simulink model "SF017A_HiLoadStallLimr"  (R2013b)
settings: Solver=FixedStepDiscrete  StartTime=0.0  StopTime=1  FixedStep=.002  RelTol=1e-3
values from neighbouring files (symbols this model uses):
  ARCHGLBPRM_2MILLISEC_SEC_F32 = DataDict.Constant    [SF017A_HiLoadStallLimr_DataDict.m]
  HiLoadStallLimrMotVelMgnThd = DataDict.Calibration    [SF017A_HiLoadStallLimr_DataDict.m]
  HiLoadStallLimrStallMotTqCmdLimY = DataDict.Calibration    [SF017A_HiLoadStallLimr_DataDict.m]
  HiLoadStallLimrStallMotTqLimSlewRate = DataDict.Calibration    [SF017A_HiLoadStallLimr_DataDict.m]
  SYSGLBPRM_MOTTQCMDHILIM_MOTNWTMTR_F32 = DataDict.Constant    [SF017A_HiLoadStallLimr_DataDict.m]
libraries: Fil x2, FixdToFloat x2, NxtrLim x2, simulink x1, FloatToFixd x1, LnrIntrpn x1
settings Model: Creator=qzwc4r  LastModifiedBy=qzwc4r
settings DataIOCC: LimitDataPoints=off  SaveFormat=Structure  ReturnWorkspaceOutputs=on
settings OptimizationCC: BlockReduction=off  InlineParams=on  ZeroExternalMemoryAtStartup=off  ZeroInternalMemoryAtStartup=off  OptimizeModelRefInitCode=on  LifeSpan=1
settings DebuggingCC: SignalInfNanChecking=error  SignalRangeChecking=warning  UnderspecifiedInitializationDetection=Simplified  SolverPrmCheckMsg=error  InheritedTsInSrcMsg=error  DiscreteInheritContinuousMsg=error  SingleTaskRateTransMsg=error  TasksWithSamePriorityMsg=error  SigSpecEnsureSampleTimeMsg=error  CheckMatrixSingularityMsg=error  IntegerOverflowMsg=error  ParameterUnderflowMsg=error  ParameterPrecisionLossMsg=error  ParameterTunabilityLossMsg=error  FixptConstUnderflowMsg=warning  FixptConstOverflowMsg=warning  VectorMatrixConversionMsg=error  SignalLabelMismatchMsg=error  UnconnectedInputMsg=error  UnconnectedOutputMsg=error  UnconnectedLineMsg=error  SFcnCompatibilityMsg=error  UniqueDataStoreMsg=warning  BusObjectLabelMismatch=error  RootOutportRequireBusObject=error  AssertControl=DisableAll  ModelReferenceIOMsg=error  ModelReferenceVersionMismatchMessage=warning  ModelReferenceIOMismatchMessage=error  ModelReferenceCSMismatchMessage=warning  ModelReferenceDataLoggingMessage=error  StateNameClashWarn=warning  StrictBusMsg=ErrorOnBusTreatedAsVector  NonBusSignalsTreatedAsBus=error  SFUnexpectedBacktrackingDiag=error  SFInvalidInputDataAccessInChartInitDiag=error  SFNoUnconditionalDefaultTransitionDiag=error  SFTransitionOutsideNaturalParentDiag=error  SFUnconditionalTransitionShadowingDiag=error  SFUndirectedBroadcastEventsDiag=error
settings ModelReferenceCC: ModelReferenceNumInstancesAllowed=Single
settings RTWCC: SystemTargetFile=autosar.tlc  GenCodeOnly=on  TemplateMakefile=ert_default_tmf  Description=AUTOSAR  GenerateReport=on  ProcessScript=autosar_make_rtw_hook  LaunchReport=on
settings CodeAppCC: GenerateComments=off  IgnoreCustomStorageClasses=off  CustomSymbolStrType=$N$R$M  CustomSymbolStrBlkIO=$N$M  SimulinkBlockComments=off
settings STFCustomTargetCC: ParMdlRefBuildCompliant=on  CompOptLevelCompliant=on  IncludeMdlTerminateFcn=off  CombineOutputUpdateFcns=on  SuppressErrorStatus=on  ERTFirstTimeCompliant=on  ERTCustomFileBanners=on  SupportNonFinite=off  SupportComplex=off  SupportContinuousTime=off  SupportNonInlinedSFcns=off  MATLABClassNameForMDSCustomization=Simulink.SoftwareTarget.ERTCustomization  AutosarCompliant=on  GRTInterface=off  SystemTargetFile=autosar.tlc
settings ERTTargetCC: CodeReplacementLibrary=ANSI_C  ConcurrentExecutionCompliant=off  IncludeMdlTerminateFcn=off  SuppressErrorStatus=on  SupportNonFinite=off  SupportComplex=off  ModelStepFunctionPrototypeControlCompliant=off  CPPClassGenCompliant=off  AutosarCompliant=on  InlinedParameterPlacement=NonHierarchical  ERTCustomFileTemplate=example_file_process.tlc  EnableUserReplacementTypes=on

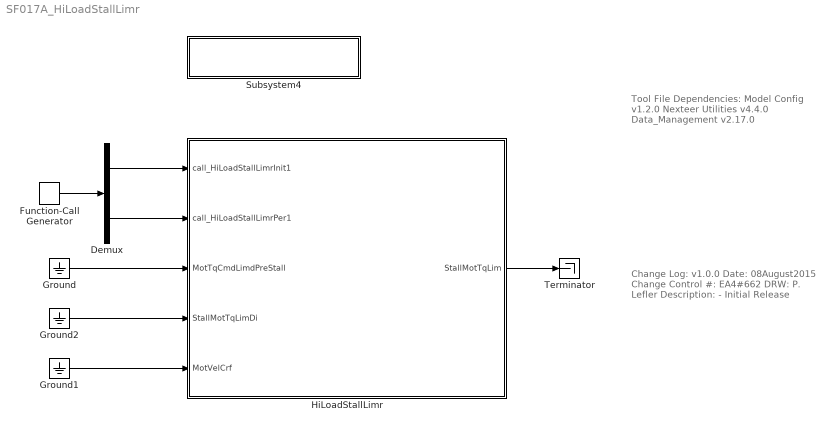
== system SF017A_HiLoadStallLimr ==
  note: Tool File Dependencies:
      |
      | Model Config v1.2.0
      | Nexteer Utilities v4.4.0
      | Data_Management v2.17.0
  note: Change Log:
      |
      | v1.0.0
      | Date: 08August2015
      | Change Control #: EA4#662
      | DRW: P. Lefler
      | Description:
      | - Initial Release
  Demux : Demux  Outputs=2
  Function-Call Generator : simulink/Ports & Subsystems/Function-Call Generator  sample_time=Ts  numberOfIterations=1
  Ground : Ground
  Ground1 : Ground
  Ground2 : Ground
  HiLoadStallLimr : Subsystem
  Subsystem4 : Subsystem  Description=|  mask(Copyright Information){none=on}
      | Copyright info block.                                               
      |                                                                     
      | Place copyright information at the top of every subsystem in design.
      mask prompts: none "No parameters"
      mask help: Place copyright information at the top of every subsystem in design.
      mask Display:
      | NxtrConf = 'Nexteer Confidential';
      | 
      | sys = bdroot; %handle for the current model ("system")
      | first = get_param(sys,'Created');
      | first = first(end-3:end);  %year is last four digits
      | 
      | last = get_param(sys,'LastModifiedDate');
      | if isempty(last)
      |     last = datestr(now,'yyyy');
      | else
      |     last = last(end-3:end);
      | end
      | 
      | if strcmp(first,last)
      |     fprintf('%s\nCopyright  %s Nexteer',NxtrConf,first);
      | else
      |     fprintf('%s\n%s%s-%s Nexteer',NxtrConf,char(169),first,last);
      | end
  Terminator : Terminator
  wires:
  Demux/1 -> HiLoadStallLimr/1(call_HiLoadStallLimrInit1)
  Demux/2 -> HiLoadStallLimr/2(call_HiLoadStallLimrPer1)
  Function-Call Generator/1 -> Demux/1
  Ground2/1 -> HiLoadStallLimr/4(StallMotTqLimDi)
  Ground/1 -> HiLoadStallLimr/3(MotTqCmdLimdPreStall)
  Ground1/1 -> HiLoadStallLimr/5(MotVelCrf)
  HiLoadStallLimr/1(StallMotTqLim) -> Terminator/1

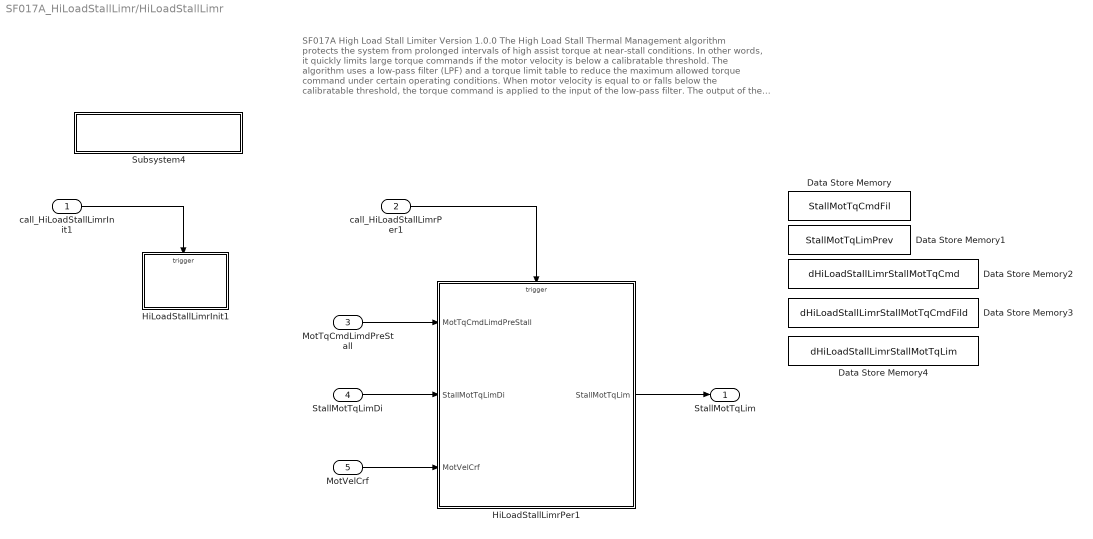
== system SF017A_HiLoadStallLimr/HiLoadStallLimr ==
  note: SF017A High Load Stall Limiter
      | Version 1.0.0
      |
      | The High Load Stall Thermal Management algorithm protects the system from prolonged intervals of high
      | assist torque at near-stall conditions. In other words, it quickly limits large torque commands if the motor
      | velocity is below a calibratable threshold.
      |      The algorithm uses a low-pass filter (LPF) and a torque limit table to reduce the maximum allowed torque
      | command under certain operating conditions. When motor velocity is equal to or falls below the calibratable
      | threshold, the torque command is applied to the input of the low-pass filter. The output of the filter ramps up
      | and indexes into the torque limit table. The output of this table is the maximum allowed torque command. A
      | slew limit calibration governs the transition rate of the table output.
  call_HiLoadStallLimrInit1 : Inport
  call_HiLoadStallLimrPer1 : Inport  Port=2
  MotTqCmdLimdPreStall : Inport  Port=3
  StallMotTqLimDi : Inport  Port=4
  MotVelCrf : Inport  Port=5
  Data Store Memory : DataStoreMemory  DataStoreName=StallMotTqCmdFil  ReadBeforeWriteMsg=warning  WriteAfterWriteMsg=warning  WriteAfterReadMsg=warning  InitialValue=[]  StateMustResolveToSignalObject=on
  Data Store Memory1 : DataStoreMemory  DataStoreName=StallMotTqLimPrev  ReadBeforeWriteMsg=warning  WriteAfterWriteMsg=warning  WriteAfterReadMsg=warning  InitialValue=[]  StateMustResolveToSignalObject=on
  Data Store Memory2 : DataStoreMemory  DataStoreName=dHiLoadStallLimrStallMotTqCmd  ReadBeforeWriteMsg=warning  WriteAfterWriteMsg=warning  WriteAfterReadMsg=warning  StateMustResolveToSignalObject=on
  Data Store Memory3 : DataStoreMemory  DataStoreName=dHiLoadStallLimrStallMotTqCmdFild  ReadBeforeWriteMsg=warning  WriteAfterWriteMsg=warning  WriteAfterReadMsg=warning  StateMustResolveToSignalObject=on
  Data Store Memory4 : DataStoreMemory  DataStoreName=dHiLoadStallLimrStallMotTqLim  ReadBeforeWriteMsg=warning  WriteAfterWriteMsg=warning  WriteAfterReadMsg=warning  StateMustResolveToSignalObject=on
  HiLoadStallLimrInit1 : Subsystem  TreatAsAtomicUnit=on
  HiLoadStallLimrPer1 : Subsystem  TreatAsAtomicUnit=on
  Subsystem4 : Subsystem  Description=|  mask(Copyright Information){none=on}
      | Copyright info block.                                               
      |                                                                     
      | Place copyright information at the top of every subsystem in design.
      mask prompts: none "No parameters"
      mask help: Place copyright information at the top of every subsystem in design.
      mask Display:
      | NxtrConf = 'Nexteer Confidential';
      | 
      | sys = bdroot; %handle for the current model ("system")
      | first = get_param(sys,'Created');
      | first = first(end-3:end);  %year is last four digits
      | 
      | last = get_param(sys,'LastModifiedDate');
      | if isempty(last)
      |     last = datestr(now,'yyyy');
      | else
      |     last = last(end-3:end);
      | end
      | 
      | if strcmp(first,last)
      |     fprintf('%s\nCopyright  %s Nexteer',NxtrConf,first);
      | else
      |     fprintf('%s\n%s%s-%s Nexteer',NxtrConf,char(169),first,last);
      | end
  StallMotTqLim : Outport
  wires:
  MotTqCmdLimdPreStall/1 -> HiLoadStallLimrPer1/1(MotTqCmdLimdPreStall)
  MotVelCrf/1 -> HiLoadStallLimrPer1/3(MotVelCrf)
  StallMotTqLimDi/1 -> HiLoadStallLimrPer1/2(StallMotTqLimDi)
  HiLoadStallLimrPer1/1(StallMotTqLim) -> StallMotTqLim/1
  call_HiLoadStallLimrPer1/1 -> HiLoadStallLimrPer1/Trigger
  call_HiLoadStallLimrInit1/1 -> HiLoadStallLimrInit1/Trigger

== system SF017A_HiLoadStallLimr/Subsystem4 ==

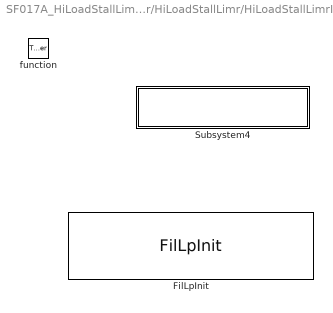
== system SF017A_HiLoadStallLimr/HiLoadStallLimr/HiLoadStallLimrInit1 ==
  function : TriggerPort  TriggerType=function-call
  FilLpInit : Fil/FilLpInit  Ic=0  Ts=ARCHGLBPRM_2MILLISEC_SEC_F32  Freq=HiLoadStallLimrMotTqCmdFilFrq  StVar=StallMotTqCmdFil
  Subsystem4 : Subsystem  Description=|  mask(Copyright Information){none=on}
      | Copyright info block.                                               
      |                                                                     
      | Place copyright information at the top of every subsystem in design.
      mask prompts: none "No parameters"
      mask help: Place copyright information at the top of every subsystem in design.
      mask Display:
      | NxtrConf = 'Nexteer Confidential';
      | 
      | sys = bdroot; %handle for the current model ("system")
      | first = get_param(sys,'Created');
      | first = first(end-3:end);  %year is last four digits
      | 
      | last = get_param(sys,'LastModifiedDate');
      | if isempty(last)
      |     last = datestr(now,'yyyy');
      | else
      |     last = last(end-3:end);
      | end
      | 
      | if strcmp(first,last)
      |     fprintf('%s\nCopyright  %s Nexteer',NxtrConf,first);
      | else
      |     fprintf('%s\n%s%s-%s Nexteer',NxtrConf,char(169),first,last);
      | end

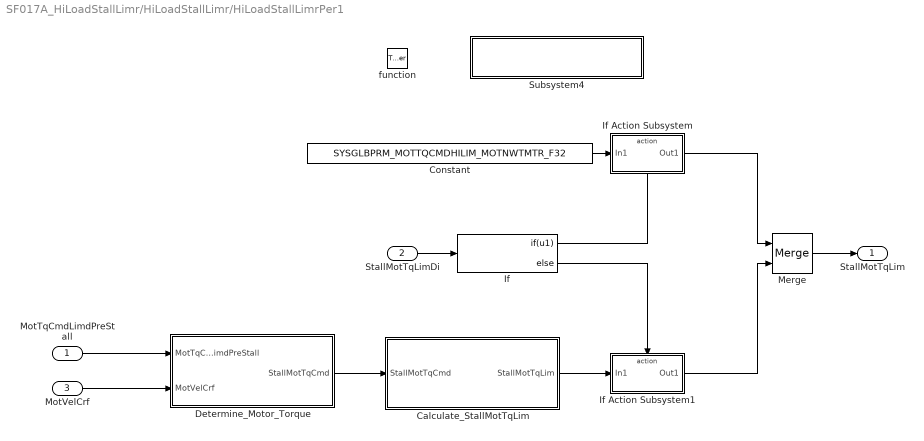
== system SF017A_HiLoadStallLimr/HiLoadStallLimr/HiLoadStallLimrPer1 ==
  MotTqCmdLimdPreStall : Inport
  StallMotTqLimDi : Inport  Port=2
  MotVelCrf : Inport  Port=3
  function : TriggerPort  TriggerType=function-call
  Calculate_StallMotTqLim : Subsystem
  Constant : Constant  Value=SYSGLBPRM_MOTTQCMDHILIM_MOTNWTMTR_F32
  Determine_Motor_Torque : Subsystem
  If : If  IfExpression=u1
  If Action Subsystem : Subsystem  TreatAsAtomicUnit=on
  If Action Subsystem1 : Subsystem  TreatAsAtomicUnit=on
  Merge : Merge
  Subsystem4 : Subsystem  Description=|  mask(Copyright Information){none=on}
      | Copyright info block.                                               
      |                                                                     
      | Place copyright information at the top of every subsystem in design.
      mask prompts: none "No parameters"
      mask help: Place copyright information at the top of every subsystem in design.
      mask Display:
      | NxtrConf = 'Nexteer Confidential';
      | 
      | sys = bdroot; %handle for the current model ("system")
      | first = get_param(sys,'Created');
      | first = first(end-3:end);  %year is last four digits
      | 
      | last = get_param(sys,'LastModifiedDate');
      | if isempty(last)
      |     last = datestr(now,'yyyy');
      | else
      |     last = last(end-3:end);
      | end
      | 
      | if strcmp(first,last)
      |     fprintf('%s\nCopyright  %s Nexteer',NxtrConf,first);
      | else
      |     fprintf('%s\n%s%s-%s Nexteer',NxtrConf,char(169),first,last);
      | end
  StallMotTqLim : Outport
  wires:
  MotTqCmdLimdPreStall/1 -> Determine_Motor_Torque/1(MotTqCmdLimdPreStall)
  MotVelCrf/1 -> Determine_Motor_Torque/2(MotVelCrf)
  Determine_Motor_Torque/1(StallMotTqCmd) -> Calculate_StallMotTqLim/1(StallMotTqCmd)
  StallMotTqLimDi/1 -> If/1
  If/1 -> If Action Subsystem/Action
  Constant/1 -> If Action Subsystem/1(In1)
  If/2 -> If Action Subsystem1/Action
  Calculate_StallMotTqLim/1(StallMotTqLim) -> If Action Subsystem1/1(In1)
  Merge/1 -> StallMotTqLim/1
  If Action Subsystem/1(Out1) -> Merge/1
  If Action Subsystem1/1(Out1) -> Merge/2

== system SF017A_HiLoadStallLimr/HiLoadStallLimr/Subsystem4 ==

== system SF017A_HiLoadStallLimr/HiLoadStallLimr/HiLoadStallLimrInit1/Subsystem4 ==

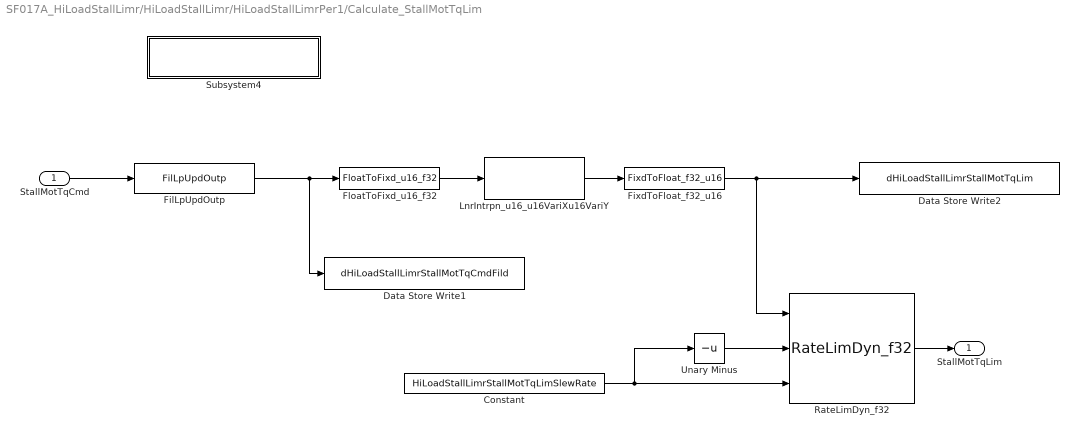
== system SF017A_HiLoadStallLimr/HiLoadStallLimr/HiLoadStallLimrPer1/Calculate_StallMotTqLim ==
  StallMotTqCmd : Inport
  Constant : Constant  Value=HiLoadStallLimrStallMotTqLimSlewRate
  Data Store Write1 : DataStoreWrite  DataStoreName=dHiLoadStallLimrStallMotTqCmdFild
  Data Store Write2 : DataStoreWrite  DataStoreName=dHiLoadStallLimrStallMotTqLim
  FilLpUpdOutp : Fil/FilLpUpdOutp  StVar=StallMotTqCmdFil
      settings: AttributesFormatString=StVar: %<StVar>
  FixdToFloat_f32_u16 : FixdToFloat/FixdToFloat_f32_u16  Param1=8
  FloatToFixd_u16_f32 : FloatToFixd/FloatToFixd_u16_f32  Param1=8
  LnrIntrpn_u16_u16VariXu16VariY : LnrIntrpn/LnrIntrpn_u16_u16VariXu16VariY  XTbl=HiLoadStallLimrStallMotTqCmdLimX  YTbl=HiLoadStallLimrStallMotTqCmdLimY
      settings: AttributesFormatString=Lnr ( u16VariX , u16VariY )
  RateLimDyn_f32 : NxtrLim/RateLimDyn_f32  StVar=StallMotTqLimPrev  Ts=ARCHGLBPRM_2MILLISEC_SEC_F32
      settings: AttributesFormatString=StVar: %<StVar>
  Subsystem4 : Subsystem  Description=|  mask(Copyright Information){none=on}
      | Copyright info block.                                               
      |                                                                     
      | Place copyright information at the top of every subsystem in design.
      mask prompts: none "No parameters"
      mask help: Place copyright information at the top of every subsystem in design.
      mask Display:
      | NxtrConf = 'Nexteer Confidential';
      | 
      | sys = bdroot; %handle for the current model ("system")
      | first = get_param(sys,'Created');
      | first = first(end-3:end);  %year is last four digits
      | 
      | last = get_param(sys,'LastModifiedDate');
      | if isempty(last)
      |     last = datestr(now,'yyyy');
      | else
      |     last = last(end-3:end);
      | end
      | 
      | if strcmp(first,last)
      |     fprintf('%s\nCopyright  %s Nexteer',NxtrConf,first);
      | else
      |     fprintf('%s\n%s%s-%s Nexteer',NxtrConf,char(169),first,last);
      | end
  Unary Minus : UnaryMinus
  StallMotTqLim : Outport
  wires:
  StallMotTqCmd/1 -> FilLpUpdOutp/1
  LnrIntrpn_u16_u16VariXu16VariY/1 -> FixdToFloat_f32_u16/1
  RateLimDyn_f32/1 -> StallMotTqLim/1
  FixdToFloat_f32_u16/1 -> Data Store Write2/1, RateLimDyn_f32/1
  FloatToFixd_u16_f32/1 -> LnrIntrpn_u16_u16VariXu16VariY/1
  Constant/1 -> RateLimDyn_f32/3, Unary Minus/1
  Unary Minus/1 -> RateLimDyn_f32/2
  FilLpUpdOutp/1 -> Data Store Write1/1, FloatToFixd_u16_f32/1

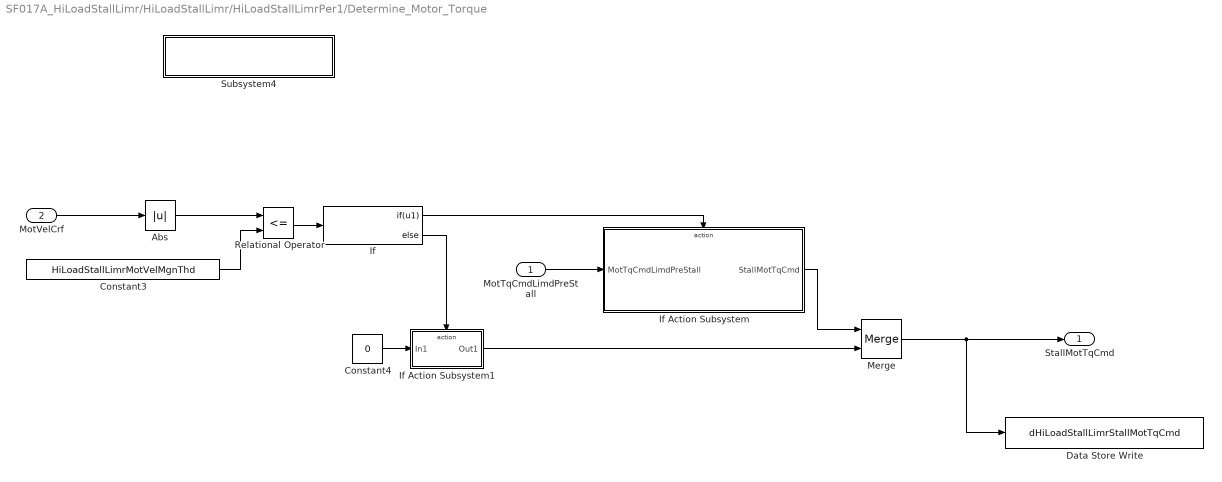
== system SF017A_HiLoadStallLimr/HiLoadStallLimr/HiLoadStallLimrPer1/Determine_Motor_Torque ==
  MotTqCmdLimdPreStall : Inport
  MotVelCrf : Inport  Port=2
  Abs : Abs
  Constant3 : Constant  Value=HiLoadStallLimrMotVelMgnThd
  Constant4 : Constant  Value=0  OutDataTypeStr=single
  Data Store Write : DataStoreWrite  DataStoreName=dHiLoadStallLimrStallMotTqCmd
  If : If  IfExpression=u1
  If Action Subsystem : Subsystem  TreatAsAtomicUnit=on
  If Action Subsystem1 : Subsystem  TreatAsAtomicUnit=on
  Merge : Merge
  Relational Operator : RelationalOperator  Operator=<=  OutDataTypeStr=boolean
  Subsystem4 : Subsystem  Description=|  mask(Copyright Information){none=on}
      | Copyright info block.                                               
      |                                                                     
      | Place copyright information at the top of every subsystem in design.
      mask prompts: none "No parameters"
      mask help: Place copyright information at the top of every subsystem in design.
      mask Display:
      | NxtrConf = 'Nexteer Confidential';
      | 
      | sys = bdroot; %handle for the current model ("system")
      | first = get_param(sys,'Created');
      | first = first(end-3:end);  %year is last four digits
      | 
      | last = get_param(sys,'LastModifiedDate');
      | if isempty(last)
      |     last = datestr(now,'yyyy');
      | else
      |     last = last(end-3:end);
      | end
      | 
      | if strcmp(first,last)
      |     fprintf('%s\nCopyright  %s Nexteer',NxtrConf,first);
      | else
      |     fprintf('%s\n%s%s-%s Nexteer',NxtrConf,char(169),first,last);
      | end
  StallMotTqCmd : Outport
  wires:
  MotVelCrf/1 -> Abs/1
  Abs/1 -> Relational Operator/1
  Constant3/1 -> Relational Operator/2
  Relational Operator/1 -> If/1
  If/1 -> If Action Subsystem/Action
  If/2 -> If Action Subsystem1/Action
  MotTqCmdLimdPreStall/1 -> If Action Subsystem/1(MotTqCmdLimdPreStall)
  Constant4/1 -> If Action Subsystem1/1(In1)
  If Action Subsystem/1(StallMotTqCmd) -> Merge/1
  If Action Subsystem1/1(Out1) -> Merge/2
  Merge/1 -> Data Store Write/1, StallMotTqCmd/1

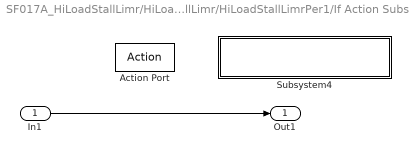
== system SF017A_HiLoadStallLimr/HiLoadStallLimr/HiLoadStallLimrPer1/If Action Subsystem ==
  In1 : Inport
  Action Port : ActionPort  ActionType=then
  Subsystem4 : Subsystem  Description=|  mask(Copyright Information){none=on}
      | Copyright info block.                                               
      |                                                                     
      | Place copyright information at the top of every subsystem in design.
      mask prompts: none "No parameters"
      mask help: Place copyright information at the top of every subsystem in design.
      mask Display:
      | NxtrConf = 'Nexteer Confidential';
      | 
      | sys = bdroot; %handle for the current model ("system")
      | first = get_param(sys,'Created');
      | first = first(end-3:end);  %year is last four digits
      | 
      | last = get_param(sys,'LastModifiedDate');
      | if isempty(last)
      |     last = datestr(now,'yyyy');
      | else
      |     last = last(end-3:end);
      | end
      | 
      | if strcmp(first,last)
      |     fprintf('%s\nCopyright  %s Nexteer',NxtrConf,first);
      | else
      |     fprintf('%s\n%s%s-%s Nexteer',NxtrConf,char(169),first,last);
      | end
  Out1 : Outport
  wires:
  In1/1 -> Out1/1

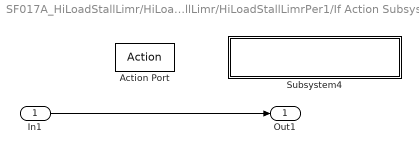
== system SF017A_HiLoadStallLimr/HiLoadStallLimr/HiLoadStallLimrPer1/If Action Subsystem1 ==
  In1 : Inport
  Action Port : ActionPort  ActionType=else
  Subsystem4 : Subsystem  Description=|  mask(Copyright Information){none=on}
      | Copyright info block.                                               
      |                                                                     
      | Place copyright information at the top of every subsystem in design.
      mask prompts: none "No parameters"
      mask help: Place copyright information at the top of every subsystem in design.
      mask Display:
      | NxtrConf = 'Nexteer Confidential';
      | 
      | sys = bdroot; %handle for the current model ("system")
      | first = get_param(sys,'Created');
      | first = first(end-3:end);  %year is last four digits
      | 
      | last = get_param(sys,'LastModifiedDate');
      | if isempty(last)
      |     last = datestr(now,'yyyy');
      | else
      |     last = last(end-3:end);
      | end
      | 
      | if strcmp(first,last)
      |     fprintf('%s\nCopyright  %s Nexteer',NxtrConf,first);
      | else
      |     fprintf('%s\n%s%s-%s Nexteer',NxtrConf,char(169),first,last);
      | end
  Out1 : Outport
  wires:
  In1/1 -> Out1/1

== system SF017A_HiLoadStallLimr/HiLoadStallLimr/HiLoadStallLimrPer1/Subsystem4 ==

== system SF017A_HiLoadStallLimr/HiLoadStallLimr/HiLoadStallLimrPer1/Calculate_StallMotTqLim/Subsystem4 ==

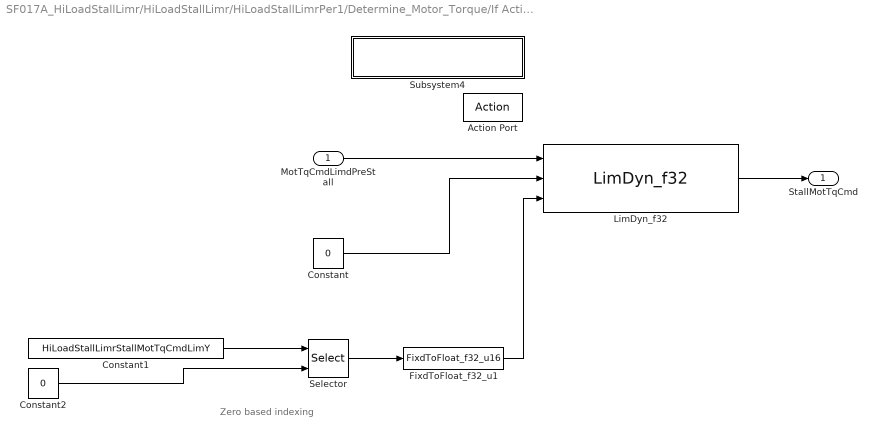
== system SF017A_HiLoadStallLimr/HiLoadStallLimr/HiLoadStallLimrPer1/Determine_Motor_Torque/If Action Subsystem ==
  note: Zero based indexing
  MotTqCmdLimdPreStall : Inport
  Action Port : ActionPort  ActionType=then
  Constant : Constant  Value=0  OutDataTypeStr=single
  Constant1 : Constant  Value=HiLoadStallLimrStallMotTqCmdLimY
  Constant2 : Constant  Value=0  OutDataTypeStr=uint16
  FixdToFloat_f32_u1 : FixdToFloat/FixdToFloat_f32_u16  Param1=8
  LimDyn_f32 : NxtrLim/LimDyn_f32
  Selector : Selector  IndexMode=Zero-based  IndexOptions=Index vector (port)  Indices=[1 3]  OutputSizes=1
  Subsystem4 : Subsystem  Description=|  mask(Copyright Information){none=on}
      | Copyright info block.                                               
      |                                                                     
      | Place copyright information at the top of every subsystem in design.
      mask prompts: none "No parameters"
      mask help: Place copyright information at the top of every subsystem in design.
      mask Display:
      | NxtrConf = 'Nexteer Confidential';
      | 
      | sys = bdroot; %handle for the current model ("system")
      | first = get_param(sys,'Created');
      | first = first(end-3:end);  %year is last four digits
      | 
      | last = get_param(sys,'LastModifiedDate');
      | if isempty(last)
      |     last = datestr(now,'yyyy');
      | else
      |     last = last(end-3:end);
      | end
      | 
      | if strcmp(first,last)
      |     fprintf('%s\nCopyright  %s Nexteer',NxtrConf,first);
      | else
      |     fprintf('%s\n%s%s-%s Nexteer',NxtrConf,char(169),first,last);
      | end
  StallMotTqCmd : Outport
  wires:
  MotTqCmdLimdPreStall/1 -> LimDyn_f32/1
  Constant/1 -> LimDyn_f32/2
  Constant2/1 -> Selector/2
  Selector/1 -> FixdToFloat_f32_u1/1
  LimDyn_f32/1 -> StallMotTqCmd/1
  Constant1/1 -> Selector/1
  FixdToFloat_f32_u1/1 -> LimDyn_f32/3

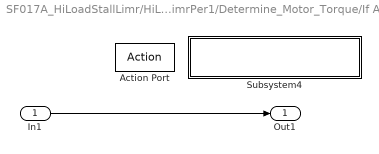
== system SF017A_HiLoadStallLimr/HiLoadStallLimr/HiLoadStallLimrPer1/Determine_Motor_Torque/If Action Subsystem1 ==
  In1 : Inport
  Action Port : ActionPort  ActionType=else
  Subsystem4 : Subsystem  Description=|  mask(Copyright Information){none=on}
      | Copyright info block.                                               
      |                                                                     
      | Place copyright information at the top of every subsystem in design.
      mask prompts: none "No parameters"
      mask help: Place copyright information at the top of every subsystem in design.
      mask Display:
      | NxtrConf = 'Nexteer Confidential';
      | 
      | sys = bdroot; %handle for the current model ("system")
      | first = get_param(sys,'Created');
      | first = first(end-3:end);  %year is last four digits
      | 
      | last = get_param(sys,'LastModifiedDate');
      | if isempty(last)
      |     last = datestr(now,'yyyy');
      | else
      |     last = last(end-3:end);
      | end
      | 
      | if strcmp(first,last)
      |     fprintf('%s\nCopyright  %s Nexteer',NxtrConf,first);
      | else
      |     fprintf('%s\n%s%s-%s Nexteer',NxtrConf,char(169),first,last);
      | end
  Out1 : Outport
  wires:
  In1/1 -> Out1/1

== system SF017A_HiLoadStallLimr/HiLoadStallLimr/HiLoadStallLimrPer1/Determine_Motor_Torque/Subsystem4 ==

== system SF017A_HiLoadStallLimr/HiLoadStallLimr/HiLoadStallLimrPer1/If Action Subsystem/Subsystem4 ==

== system SF017A_HiLoadStallLimr/HiLoadStallLimr/HiLoadStallLimrPer1/If Action Subsystem1/Subsystem4 ==

== system SF017A_HiLoadStallLimr/HiLoadStallLimr/HiLoadStallLimrPer1/Determine_Motor_Torque/If Action Subsystem/Subsystem4 ==

== system SF017A_HiLoadStallLimr/HiLoadStallLimr/HiLoadStallLimrPer1/Determine_Motor_Torque/If Action Subsystem1/Subsystem4 ==
